simulink model "gm_external_state_machine"  (R2021a)
settings: Solver=FixedStepDiscrete  StartTime=0.0  StopTime=200*t_ADC  RelTol=1e-3
undefined symbols (not defined in the file or in its folder): A, IB, id_ref, iq_ref, ix_ref, iy_ref, lambda_d, lambda_q, lambda_u, lambda_x, lambda_y, Ld_over_LB, Lq_over_LB, n_rpm, omega_m, omegaB, p, psi_pm_over_psiB, Rs_over_ZB, t_ADC, t_clock, Ts_times_ZB_over_Ld, Ts_times_ZB_over_Lq, Ts_times_ZB_over_Lx, Ts_times_ZB_over_Ly, v_dc, VB
libraries: nesl_utility x38, fl_lib x30, simulink x19, ee_lib x14, hdlsllib x4, spsAlphaBetaZerotodq0Lib x1
(part 4 of 4)

== matlab function gm_external_state_machine/MATLAB Function ==
  data: u input; G_opt output; opt_idx output
function [G_opt,opt_idx] = fcn(u)
%#codegen
G = [0,1,0,1,0,1,0,1,0,1,0,1;1,0,1,0,0,1,1,0,1,0,0,1;1,0,1,0,0,1,1,0,1,0,0,1;0,1,1,0,0,1,1,0,1,0,0,1;1,0,1,0,0,1,1,0,1,0,0,1;0,1,1,0,0,1,1,0,1,0,0,1;1,0,1,0,0,1,1,0,1,0,0,1;0,1,1,0,0,1,1,0,1,0,0,1;1,0,1,0,0,1,1,0,1,0,0,1;0,1,1,0,0,1,1,0,1,0,0,1;1,0,1,0,0,1,1,0,1,0,0,1;0,1,1,0,0,1,1,0,1,0,0,1;1,0,1,0,0,1,1,0,1,0,0,1;0,1,1,0,0,1,1,0,1,0,0,1;1,0,1,0,0,1,1,0,1,0,0,1;0,1,1,0,0,1,1,0,1,0,0,1;1,0,1,0,0,1,1,0,1,0,0,1;0,1,1,0,0,1,1,0,1,0,0,1;1,0,1,0,0,1,1,0,1,0,0,1;0,1,1,0,0,1,1,0,1,0,0,1;1,0,1,0,0,1,1,0,1,0,0,1;0,1,1,0,0,1,1,0,1,0,0,1;1,0,1,0,0,1,1,0,1,0,0,1;0,1,1,0,0,1,1,0,1,0,0,1;1,0,1,0,0,1,1,0,1,0,0,1;0,1,1,0,0,1,1,0,1,0,0,1;1,0,1,0,0,1,1,0,1,0,0,1;0,1,1,0,0,1,1,0,1,0,0,1;1,0,1,0,0,1,1,0,1,0,0,1;0,1,1,0,0,1,1,0,1,0,0,1;1,0,1,0,0,1,1,0,1,0,0,1;0,1,1,0,0,1,1,0,1,0,0,1;1,0,1,0,0,1,1,0,1,0,0,1;0,1,1,0,0,1,1,0,1,0,0,1;1,0,1,0,0,1,1,0,1,0,0,1;0,1,1,0,0,1,1,0,1,0,0,1;1,0,1,0,0,1,1,0,1,0,0,1;0,1,1,0,0,1,1,0,1,0,0,1;1,0,1,0,0,1,1,0,1,0,0,1;0,1,1,0,0,1,1,0,1,0,0,1;1,0,1,0,0,1,1,0,1,0,0,1;0,1,1,0,0,1,1,0,1,0,0,1;1,0,1,0,0,1,1,0,1,0,0,1;0,1,1,0,0,1,1,0,1,0,0,1;1,0,1,0,0,1,1,0,1,0,0,1;0,1,1,0,0,1,1,0,1,0,0,1;1,0,1,0,0,1,1,0,1,0,0,1;0,1,1,0,0,1,1,0,1,0,0,1;1,0,1,0,0,1,1,0,1,0,0,1;0,1,1,0,0,1,1,0,1,0,0,1;1,0,1,0,0,1,1,0,1,0,0,1;0,1,1,0,0,1,1,0,1,0,0,1;1,0,1,0,0,1,1,0,1,0,0,1;0,1,1,0,0,1,1,0,1,0,0,1;1,0,1,0,0,1,1,0,1,0,0,1;0,1,1,0,0,1,1,0,1,0,0,1;1,0,1,0,0,1,1,0,1,0,0,1;0,1,1,0,0,1,1,0,1,0,0,1;1,0,1,0,0,1,1,0,1,0,0,1;0,1,1,0,0,1,1,0,1,0,0,1;1,0,1,0,0,1,1,0,1,0,0,1;0,1,1,0,0,1,1,0,1,0,0,1;1,0,1,0,0,1,1,0,1,0,0,1;0,1,1,0,0,1,1,0,1,0,0,1;1,0,1,0,0,1,1,0,1,0,0,1;0,1,1,0,0,1,1,0,1,0,0,1;1,0,1,0,0,1,1,0,1,0,0,1;0,1,1,0,0,1,1,0,1,0,0,1;1,0,1,0,0,1,1,0,1,0,0,1;0,1,1,0,0,1,1,0,1,0,0,1;1,0,1,0,0,1,1,0,1,0,0,1;0,1,1,0,0,1,1,0,1,0,0,1;1,0,1,0,0,1,1,0,1,0,0,1;0,1,0,1,1,0,1,0,1,0,0,1;1,0,0,1,1,0,1,0,1,0,0,1;0,1,1,0,1,0,1,0,1,0,0,1;1,0,1,0,1,0,1,0,1,0,0,1;0,1,0,1,0,1,0,1,0,1,1,0;1,0,0,1,0,1,0,1,0,1,1,0;0,1,1,0,0,1,0,1,0,1,1,0;1,0,1,0,0,1,0,1,0,1,1,0;0,1,0,1,1,0,0,1,0,1,1,0;1,0,0,1,1,0,0,1,0,1,1,0;0,1,1,0,1,0,0,1,0,1,1,0;1,0,1,0,1,0,0,1,0,1,1,0;0,1,0,1,0,1,1,0,0,1,1,0;1,0,0,1,0,1,1,0,0,1,1,0;0,1,1,0,0,1,1,0,0,1,1,0;1,0,1,0,0,1,1,0,0,1,1,0;0,1,1,0,0,1,1,0,0,1,1,0;1,0,1,0,0,1,1,0,0,1,1,0;0,1,0,1,0,1,0,1,1,0,1,0;0,1,1,0,0,1,0,1,1,0,1,0;1,0,1,0,0,1,0,1,1,0,1,0;0,1,1,0,0,1,0,1,1,0,1,0;1,0,1,0,0,1,0,1,1,0,1,0;0,1,1,0,0,1,0,1,1,0,1,0;1,0,1,0,0,1,0,1,1,0,1,0;0,1,1,0,0,1,0,1,1,0,1,0;1,0,1,0,0,1,0,1,1,0,1,0;1,0,1,0,0,1,0,1,1,0,1,0];
idx = [0;28;28;27;28;27;28;27;28;27;28;27;28;27;28;27;28;27;28;27;28;27;28;27;28;27;28;27;28;27;28;27;28;27;28;27;28;27;28;27;28;27;28;27;28;27;28;27;28;27;28;27;28;27;28;27;28;27;28;27;28;27;28;27;28;27;28;27;28;27;28;27;28;29;30;31;32;33;34;35;36;37;38;39;40;41;42;43;44;43;44;49;51;52;51;52;51;52;51;52;52];


G_opt = G(u,:);
opt_idx = idx(u);

== matlab function gm_external_state_machine/6ph_PMSM_30deg_VSD1 ==
  data: u1 input; y1 output; u2 input; u3 input; u4 input; u5 input; u6 input; y2 output; y3 output; y4 output; y5 output; y6 output; k6 input; c6 input
function [y1,y2,y3,y4,y5,y6] = VSD_asymm_30(u1,u2,u3,u4,u5,u6,k6,c6)

A = [0 0 0 0 0 0]';

A =    k6*[1    -0.5        -0.5        sqrt(3)/2   -sqrt(3)/2  0 ;
           0    sqrt(3)/2   -sqrt(3)/2  0.5         0.5         -1;
           1    -0.5        -0.5        -sqrt(3)/2  sqrt(3)/2   0 ;
           0    -sqrt(3)/2  sqrt(3)/2   0.5         0.5         -1;
           c6   c6          c6          0           0           0 ;
           0    0           0           c6          c6          c6] * [u1 u2 u3 u4 u5 u6]';

y1 = A(1);
y2 = A(2);
y3 = A(3);
y4 = A(4);
y5 = A(5);
y6 = A(6);

== matlab function gm_external_state_machine/cost_opt/FiniteControlSetSwitchingTable ==
  settings: fimath=fimath('RoundingMethod', 'Floor','OverflowAction', 'Wrap','ProductMode', 'FullPrecision', 'SumMode', 'FullPrecision')
  data: G output
function G  = switchingTable

% -------------------------------------------------------------------
%  Generated by MATLAB on 14-Oct-2020 14:52:37
%  MATLAB version: 9.4.0.813654 (R2018a)
% -------------------------------------------------------------------
                                         

s1_v = boolean([0; 1; 0; 1; 0; 1; 0; 1; 0; 1; 0; 1; 0; 1; 0; 1; 0; 1; 0; 1; 0; ...
        1; 0; 1; 0; 1; 0; 1; 0; 1; 0; 1; 0; 1; 0; 1; 0; 1; 0; 1; 0; 1; ...
        0; 1; 0; 1; 0; 1; 0; 1; 0; 1; 0; 1; 0; 1; 0; 1; 0; 1; 0; 1; 0; ...
        1]);


s2_v = boolean([1; 0; 1; 0; 1; 0; 1; 0; 1; 0; 1; 0; 1; 0; 1; 0; 1; 0; 1; 0; 1; ...
        0; 1; 0; 1; 0; 1; 0; 1; 0; 1; 0; 1; 0; 1; 0; 1; 0; 1; 0; 1; 0; ...
        1; 0; 1; 0; 1; 0; 1; 0; 1; 0; 1; 0; 1; 0; 1; 0; 1; 0; 1; 0; 1; ...
        0]);


s3_v = boolean([0; 0; 1; 1; 0; 0; 1; 1; 0; 0; 1; 1; 0; 0; 1; 1; 0; 0; 1; 1; 0; ...
        0; 1; 1; 0; 0; 1; 1; 0; 0; 1; 1; 0; 0; 1; 1; 0; 0; 1; 1; 0; 0; ...
        1; 1; 0; 0; 1; 1; 0; 0; 1; 1; 0; 0; 1; 1; 0; 0; 1; 1; 0; 0; 1; ...
        1]);


s4_v = boolean([1; 1; 0; 0; 1; 1; 0; 0; 1; 1; 0; 0; 1; 1; 0; 0; 1; 1; 0; 0; 1; ...
        1; 0; 0; 1; 1; 0; 0; 1; 1; 0; 0; 1; 1; 0; 0; 1; 1; 0; 0; 1; 1; ...
        0; 0; 1; 1; 0; 0; 1; 1; 0; 0; 1; 1; 0; 0; 1; 1; 0; 0; 1; 1; 0; ...
        0]);


s5_v = boolean([0; 0; 0; 0; 1; 1; 1; 1; 0; 0; 0; 0; 1; 1; 1; 1; 0; 0; 0; 0; 1; ...
        1; 1; 1; 0; 0; 0; 0; 1; 1; 1; 1; 0; 0; 0; 0; 1; 1; 1; 1; 0; 0; ...
        0; 0; 1; 1; 1; 1; 0; 0; 0; 0; 1; 1; 1; 1; 0; 0; 0; 0; 1; 1; 1; ...
        1]);


s6_v = boolean([1; 1; 1; 1; 0; 0; 0; 0; 1; 1; 1; 1; 0; 0; 0; 0; 1; 1; 1; 1; 0; ...
        0; 0; 0; 1; 1; 1; 1; 0; 0; 0; 0; 1; 1; 1; 1; 0; 0; 0; 0; 1; 1; ...
        1; 1; 0; 0; 0; 0; 1; 1; 1; 1; 0; 0; 0; 0; 1; 1; 1; 1; 0; 0; 0; ...
        0]);


s7_v = boolean([0; 0; 0; 0; 0; 0; 0; 0; 1; 1; 1; 1; 1; 1; 1; 1; 0; 0; 0; 0; 0; ...
        0; 0; 0; 1; 1; 1; 1; 1; 1; 1; 1; 0; 0; 0; 0; 0; 0; 0; 0; 1; 1; ...
        1; 1; 1; 1; 1; 1; 0; 0; 0; 0; 0; 0; 0; 0; 1; 1; 1; 1; 1; 1; 1; ...
        1]);


s8_v = boolean([1; 1; 1; 1; 1; 1; 1; 1; 0; 0; 0; 0; 0; 0; 0; 0; 1; 1; 1; 1; 1; ...
        1; 1; 1; 0; 0; 0; 0; 0; 0; 0; 0; 1; 1; 1; 1; 1; 1; 1; 1; 0; 0; ...
        0; 0; 0; 0; 0; 0; 1; 1; 1; 1; 1; 1; 1; 1; 0; 0; 0; 0; 0; 0; 0; ...
        0]);


s9_v = boolean([0; 0; 0; 0; 0; 0; 0; 0; 0; 0; 0; 0; 0; 0; 0; 0; 1; 1; 1; 1; 1; ...
        1; 1; 1; 1; 1; 1; 1; 1; 1; 1; 1; 0; 0; 0; 0; 0; 0; 0; 0; 0; 0; ...
        0; 0; 0; 0; 0; 0; 1; 1; 1; 1; 1; 1; 1; 1; 1; 1; 1; 1; 1; 1; 1; ...
        1]);


s10_v = boolean([1; 1; 1; 1; 1; 1; 1; 1; 1; 1; 1; 1; 1; 1; 1; 1; 0; 0; 0; 0; 0; ...
         0; 0; 0; 0; 0; 0; 0; 0; 0; 0; 0; 1; 1; 1; 1; 1; 1; 1; 1; 1; 1; ...
         1; 1; 1; 1; 1; 1; 0; 0; 0; 0; 0; 0; 0; 0; 0; 0; 0; 0; 0; 0; 0; ...
         0]);


s11_v = boolean([0; 0; 0; 0; 0; 0; 0; 0; 0; 0; 0; 0; 0; 0; 0; 0; 0; 0; 0; 0; 0; ...
         0; 0; 0; 0; 0; 0; 0; 0; 0; 0; 0; 1; 1; 1; 1; 1; 1; 1; 1; 1; 1; ...
         1; 1; 1; 1; 1; 1; 1; 1; 1; 1; 1; 1; 1; 1; 1; 1; 1; 1; 1; 1; 1; ...
         1]);


s12_v = boolean([1; 1; 1; 1; 1; 1; 1; 1; 1; 1; 1; 1; 1; 1; 1; 1; 1; 1; 1; 1; 1; ...
         1; 1; 1; 1; 1; 1; 1; 1; 1; 1; 1; 0; 0; 0; 0; 0; 0; 0; 0; 0; 0; ...
         0; 0; 0; 0; 0; 0; 0; 0; 0; 0; 0; 0; 0; 0; 0; 0; 0; 0; 0; 0; 0; ...
         0]);
     
G = [s1_v, s2_v, s3_v, s4_v, s5_v, s6_v, s7_v, s8_v, s9_v, s10_v, s11_v, s12_v];

== matlab function gm_external_state_machine/Subsystem2/Count_f_sw ==
  data: switchNumb input fixdt(0,25,0); ss_v_old input; ss_v input; switchNumbOut output fixdt(0,25,0); bReset input
 function switchNumbOut   = Count_f_sw(switchNumb,ss_v_old,ss_v, bReset)
   %
    %% toDO
        %s
 
    %% Initialization
    Fq25    = fimath('RoundingMethod', 'Floor', 'OverflowAction', 'Wrap','ProductMode', 'FullPrecision', 'ProductWordLength', 25,'ProductFractionLength',0,'SumMode','SpecifyPrecision','SumWordLength',25,'SumFractionLength',0);

    % I need this initialization, in order that the HDL Coder and Simulink knows the size of the vectors! Without these, i will get an error!
   % idx_globalOld     = fi(1, 0, 8, 0); % Chosen position overall in the error vector
    %switchNumb = fi(0, 0, 25, 0);
    
    %% Reset the counters (similar to the THD, i will try to average the switching frequency over 20 fundamental periods. After this time, a Reset-Flag from the ARM processor will reset the counter) 
    if (bReset == true) 
        switchNumb = fi(0, 0, 25, 0);
    end
    %% Check if switching occurs. If yes count up.
    % However, dependent of the ss_v before, switching can but do not have to occure, if the previously applied ss_v keeps.

    %Use a for-loop since in VHDL i have time and can do a resource streaming
    %Even if i need 6 cycles @100MHz, since it is not able to have have
    %switching (on/off inside of 60ns), this is ok (because T_cf = 10us and
    %and switching for such a short time is not allwoed nayway, since it is
    %not worth it (too much losses).)
    for countSS=fi(1, 0, 8, 0):fi(12, 0, 8, 0) %1:12
        if (ss_v(countSS) ~= ss_v_old(countSS)) %Check if switch has changed
            switchNumb = fi(add(Fq25,switchNumb,fi(1, 0, 25, 0)),0,25,0); % +1 Increment the switch counter +1
        end
    end

    switchNumbOut = switchNumb;

 end
